simulink model "hw1"  (R2017a)
settings: Solver=VariableStepAuto  StartTime=0.0  StopTime=10.0  RelTol=1e-3
settings Model: Creator=SharPing  LastModifiedBy=SharPing

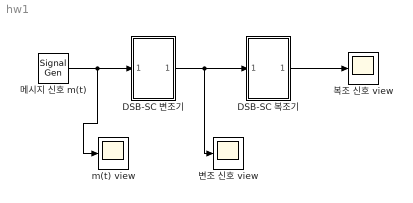
== system hw1 ==
  DSB-SC 변조기 : Subsystem
  DSB-SC 복조기 : Subsystem
  m(t) view : Scope
  메시지 신호 m(t) : SignalGenerator  WaveForm=square  Units=rad/sec
  변조 신호 view : Scope
  복조 신호 view : Scope
  wires:
  메시지 신호 m(t)/1 -> m(t) view/1, DSB-SC 변조기/1(In1)
  DSB-SC 변조기/1(Out1) -> 변조 신호 view/1, DSB-SC 복조기/1(In1)
  DSB-SC 복조기/1(Out1) -> 복조 신호 view/1

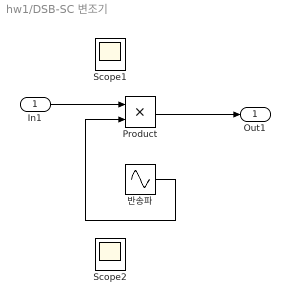
== system hw1/DSB-SC 변조기 ==
  In1 : Inport
  Product : Product
  Scope1 : Scope
  Scope2 : Scope
  반송파 : Sin  Frequency=2*pi  Phase=pi/2  SampleTime=0
  Out1 : Outport
  wires:
  Product/1 -> Out1/1
  In1/1 -> Product/1
  반송파/1 -> Product/2

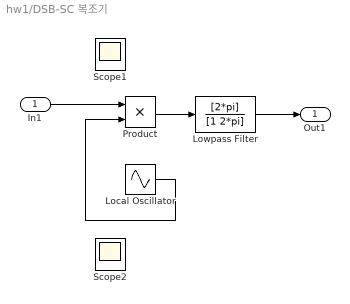
== system hw1/DSB-SC 복조기 ==
  In1 : Inport
  Local Oscillator : Sin  Frequency=2*pi  Phase=pi/2  SampleTime=0
  Lowpass Filter : TransferFcn  Numerator=[2*pi]  Denominator=[1 2*pi]
  Product : Product
  Scope1 : Scope
  Scope2 : Scope
  Out1 : Outport
  wires:
  Product/1 -> Lowpass Filter/1
  In1/1 -> Product/1
  Local Oscillator/1 -> Product/2
  Lowpass Filter/1 -> Out1/1
